simulink subsystem "Longitudinal_Acceleration_Control"  (R2021b)
settings: Solver=VariableStepAuto  StartTime=0.0  StopTime=10.0  RelTol=1e-3
settings Model: Creator=gabep  LastModifiedBy=gabep

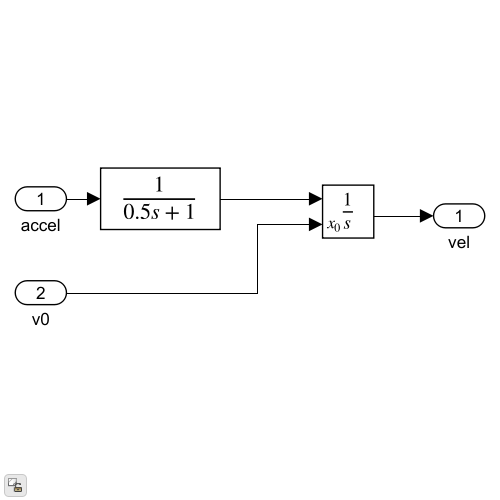
[thumbnail: Simulink's stored preview of the top-level diagram]
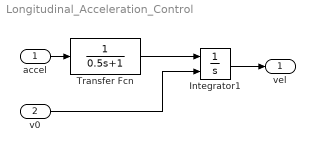
== system Longitudinal_Acceleration_Control ==
  accel : Inport
  v0 : Inport  Port=2
  Integrator1 : Integrator  InitialConditionSource=external
  Transfer Fcn : TransferFcn  Denominator=[0.5 1]
  vel : Outport
  wires:
  accel/1 -> Transfer Fcn/1
  v0/1 -> Integrator1/2
  Integrator1/1 -> vel/1
  Transfer Fcn/1 -> Integrator1/1
